simulink model "Advanced_PID_tout"  (R2023a)
settings: Solver=VariableStepAuto  StartTime=0.0  StopTime=5000  RelTol=1e-3
libraries: cstblocks x2, slpidlib x1
settings Model: Creator=Yuganshu Wadhwa  LastModifiedBy=Yuganshu Wadhwa

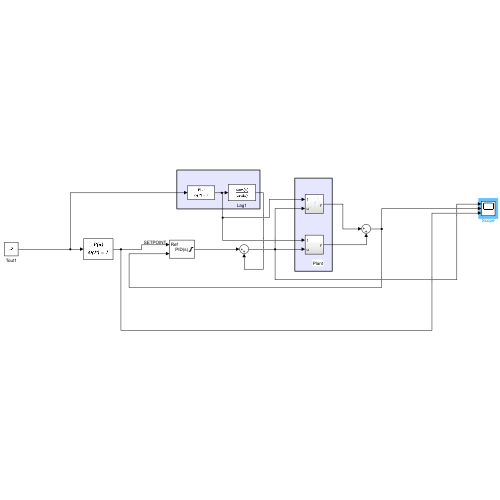
[thumbnail: Simulink's stored preview of the top-level diagram]
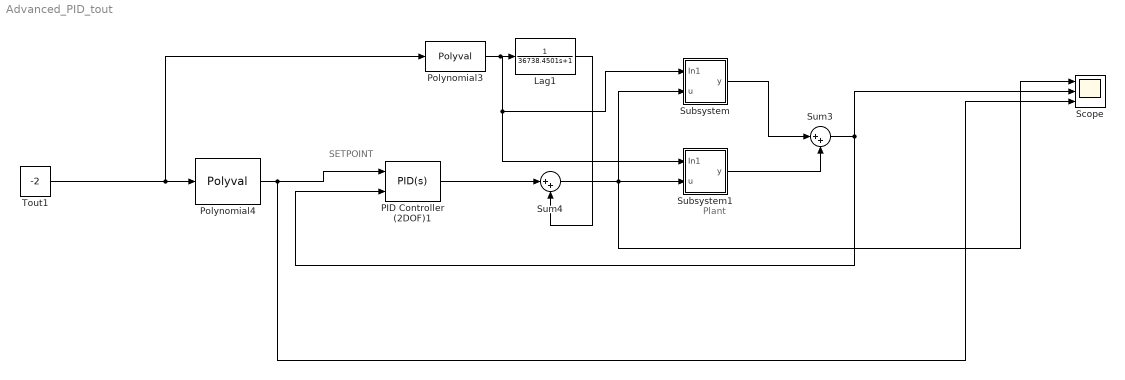
== system Advanced_PID_tout ==
  note: SETPOINT
  note: Plant
  Lag1 : TransferFcn  Denominator=[36738.4501 1]
  PID Controller (2DOF)1 : slpidlib/PID Controller (2DOF)  Controller=PID  Form=Parallel  TimeDomain=Continuous-time  UseExternalTs=off  SampleTime=-1  IntegratorMethod=Forward Euler  FilterMethod=Forward Euler  ControllerParametersSource=internal  P=1  I=1  UseKiTs=off  D=0  N=100  UseFilter=on  b=1  c=1  TunerSelectOption=Frequency Response Based  InitialConditionSource=internal  InitialConditionForIntegrator=0  InitialConditionForFilter=0  DifferentiatorICPrevScaledInput=0  ExternalReset=none  TrackingMode=off  Kt=1  LimitOutput=on  SatLimitsSource=internal  UpperSaturationLimit=100  LowerSaturationLimit=0  LinearizeAsGain=on  AntiWindupMode=none  Kb=1  LimitIntegrator=off  UpperIntegratorSaturationLimit=inf  LowerIntegratorSaturationLimit=-inf  POutMin=[]  POutMax=[]  IOutMin=[]  IOutMax=[]  DOutMin=[]  DOutMax=[]  NOutMin=[]  NOutMax=[]  bOutMin=[]  bOutMax=[]  cOutMin=[]  cOutMax=[]  SumOutMin=[]  SumOutMax=[]  SaturationOutMin=[]  SaturationOutMax=[]  PParamMin=[]  PParamMax=[]  IParamMin=[]  IParamMax=[]  DParamMin=[]  DParamMax=[]  NParamMin=[]  NParamMax=[]  bParamMin=[]  bParamMax=[]  cParamMin=[]  cParamMax=[]  KbParamMin=[]  KbParamMax=[]  KtParamMin=[]  KtParamMax=[]  KbOutMin=[]  KbOutMax=[]  KtOutMin=[]  KtOutMax=[]  IntegratorOutMin=[]  IntegratorOutMax=[]  FilterOutMin=[]  FilterOutMax=[]  SumI1OutMin=[]  SumI1OutMax=[]  SumI2OutMin=[]  SumI2OutMax=[]  SumI3OutMin=[]  SumI3OutMax=[]  SumI4OutMin=[]  SumI4OutMax=[]  SumDOutMin=[]  SumDOutMax=[]  Sum1OutMin=[]  Sum1OutMax=[]  Sum2OutMin=[]  Sum2OutMax=[]  Sum3OutMin=[]  Sum3OutMax=[]  DifferentiatorOutMin=[]  DifferentiatorOutMax=[]  FilterDiffOutCoefMin=[]  FilterDiffOutCoefMax=[]  ReciprocalOutMin=[]  ReciprocalOutMax=[]  SumDenOutMin=[]  SumDenOutMax=[]  SumNumOutMin=[]  SumNumOutMax=[]  DivideOutMin=[]  DivideOutMax=[]  UdiffTsProdOutMin=[]  UdiffTsProdOutMax=[]  NTsProdOutMin=[]  NTsProdOutMax=[]  UintegralTsProdOutMin=[]  UintegralTsProdOutMax=[]  UngainTsProdOutMin=[]  UngainTsProdOutMax=[]  ClampingZeroOutDataTypeStr=Inherit: Inherit via back propagation  ClampingZeroOutMin=[]  ClampingZeroOutMax=[]  FilterDenConstantOutDataTypeStr=Inherit: Inherit via back propagation  FilterDenConstantOutMin=[]  FilterDenConstantOutMax=[]  PCopyOutDataTypeStr=Inherit: Inherit via back propagation  PCopyOutMin=[]  PCopyOutMax=[]  NCopyOutDataTypeStr=Inherit: Inherit via back propagation  NCopyOutMin=[]  NCopyOutMax=[]  IntegratorContinuousStateAttributes=''  IntegratorStateMustResolveToSignalObject=off  IntegratorRTWStateStorageClass=Auto  FilterContinuousStateAttributes=''  FilterStateMustResolveToSignalObject=off  FilterRTWStateStorageClass=Auto  ParallelPVariant=InternalParameters  IdealPVariant=Disabled  IVariant=InternalParameters  DVariant=InternalParameters  bVariant=InternalParameters  cVariant=InternalParameters  IntegratorVariant=Continuous  SatVariant=Enabled  AWVariant=Passthrough  PCopyVariant=Disabled  TRVariant=Disabled  FdbkBlocksVariant=Forward  IdealPFdbkVariant=Disabled  SatFdbkVariant=Disabled  DerivativeFilterVariant=ContFilter  NVariant=InternalParameters  NCopyVariant=Disabled  FilterICVariant=InternalICsFilter  IntegratorICVariant=InternalICs  ExternalResetVariant=Disabled  TRSumVariant=Passthrough  SumFdbkVariant=Disabled  SumVariant=Sum_PID  TsampFilterVariant=InternalTs  TsampNgainVariant=Passthrough  TsampIntegralVariant=Disabled_SignalSpec  ExternalSaturationOutDataTypeStr=Inherit: Same as second input
  Polynomial3 : Polyval  Coefs=[ +0.5285, +0.2364, +16.302 ]
  Polynomial4 : Polyval  Coefs=[ -0.1576, 31.999 ]
  Scope : Scope  NumInputPorts=3
  Subsystem : Subsystem
  Subsystem1 : Subsystem
  Sum3 : Sum  Inputs=|++
  Sum4 : Sum  Inputs=|++
  Tout1 : Constant  Value=-2
  wires:
  Sum3/1 -> Scope/2, PID Controller (2DOF)1/2
  Subsystem/1(y) -> Sum3/1
  Polynomial4/1 -> Scope/3, PID Controller (2DOF)1/1
  Polynomial3/1 -> Subsystem/1(In1), Subsystem1/1(In1), Lag1/1
  Lag1/1 -> Sum4/2
  Tout1/1 -> Polynomial3/1, Polynomial4/1
  PID Controller (2DOF)1/1 -> Sum4/1
  Subsystem1/1(y) -> Sum3/2
  Sum4/1 -> Scope/1, Subsystem/2(u), Subsystem1/2(u)

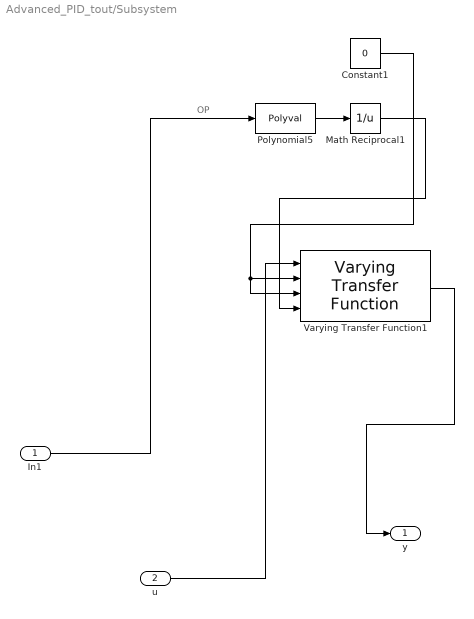
== system Advanced_PID_tout/Subsystem ==
  note: OP
  In1 : Inport
  u : Inport  Port=2
  Constant1 : Constant  Value=0
  Math Reciprocal1 : Math  Operator=reciprocal  SignedPower=on
  Polynomial5 : Polyval  Coefs=[ +511.04, -14301, +405369 ]
  Varying Transfer Function1 : cstblocks/Linear Parameter Varying/Varying Transfer Function  N=1  Feedthrough=on
  y : Outport
  wires:
  In1/1 -> Polynomial5/1
  Constant1/1 -> Varying Transfer Function1/2, Varying Transfer Function1/3
  Polynomial5/1 -> Math Reciprocal1/1
  Varying Transfer Function1/1 -> y/1
  Math Reciprocal1/1 -> Varying Transfer Function1/4
  u/1 -> Varying Transfer Function1/1

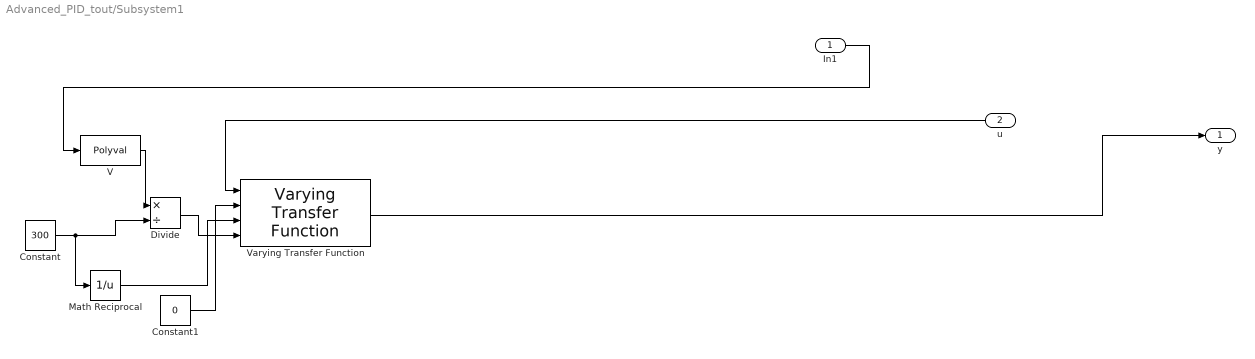
== system Advanced_PID_tout/Subsystem1 ==
  In1 : Inport
  u : Inport  Port=2
  Constant : Constant  Value=300
  Constant1 : Constant  Value=0
  Divide : Product  Inputs=*/
  Math Reciprocal : Math  Operator=reciprocal  SignedPower=on
  V : Polyval  Coefs="[  -3e-7, +8e-5, -0.0065, 0.1944 ]"
  Varying Transfer Function : cstblocks/Linear Parameter Varying/Varying Transfer Function  N=1  Feedthrough=on
  y : Outport
  wires:
  Divide/1 -> Varying Transfer Function/4
  Constant/1 -> Math Reciprocal/1, Divide/2
  Constant1/1 -> Varying Transfer Function/2
  In1/1 -> V/1
  V/1 -> Divide/1
  u/1 -> Varying Transfer Function/1
  Math Reciprocal/1 -> Varying Transfer Function/3
  Varying Transfer Function/1 -> y/1
